simulink model "test"  (R2020b)
settings: Solver=FixedStepDiscrete  StartTime=0.0  StopTime=Inf  RelTol=1e-3
libraries: rpi_blkst x2
settings Model: Creator=jacques  LastModifiedBy=jacques
settings DataIOCC: ReturnWorkspaceOutputs=off
settings OptimizationCC: EnhancedBackFolding=on  PassReuseOutputArgsAs=Individual arguments  ZeroExternalMemoryAtStartup=off  ZeroInternalMemoryAtStartup=off  OptimizeBlockOrder=speed  DifferentSizesBufferReuse=on  OptimizationCustomize=off  EfficientTunableParamExpr=on
settings DebuggingCC: ParameterTunabilityLossMsg=error
settings HardwareCC: ProdBitPerPointer=32  ProdBitPerSizeT=32  ProdBitPerPtrDiffT=32  ProdLargestAtomicInteger=Long  ProdLargestAtomicFloat=Double  ProdWordSize=32  ProdHWDeviceType=ARM Compatible->ARM 11
settings SFSimCC: MATLABDynamicMemAlloc=off
settings RTWCC: Description=RTW Embedded Coder RPI target  SystemTargetFile=ert_rpi.tlc  TemplateMakefile=ert_rpi.tmf  PostCodeGenCommand=postGenFunc(buildInfo)
settings CodeAppCC: ForceParamTrailComments=on  IgnoreCustomStorageClasses=off  OperatorAnnotations=on  SimulinkDataObjDesc=on  SFDataObjDesc=on  InsertBlockDesc=on
settings STFCustomTargetCC: TargetLangStandard=C99 (ISO)  MultiwordLength=256  ModelReferenceCompliant=off  ConcurrentExecutionCompliant=off  CombineOutputUpdateFcns=on  ERTCustomFileBanners=on  SupportNonInlinedSFcns=off  RemoveResetFunc=on  MATLABClassNameForMDSCustomization=Simulink.SoftwareTarget.ERTCustomization  CPPClassGenCompliant=off  GRTInterface=off  SystemTargetFile=ert_rpi.tlc
settings ERTTargetCC: TargetLangStandard=C99 (ISO)  ModelReferenceCompliant=off  ParMdlRefBuildCompliant=off  CompOptLevelCompliant=off  ConcurrentExecutionCompliant=off  SupportContinuousTime=on  ModelStepFunctionPrototypeControlCompliant=off  CPPClassGenCompliant=off  UseToolchainInfoCompliant=off  ExtMode=on  ExtModeMexArgs='10.211.55.9'  ERTCustomFileTemplate=ert_rpi_file_process.tlc

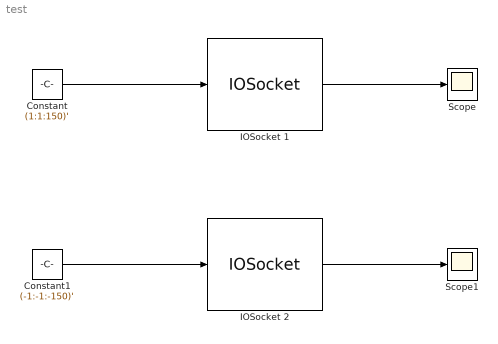
== system test ==
  Constant : Constant  Value=(1:1:150)'  SampleTime=0.05
  Constant1 : Constant  Value=(-1:-1:-150)'  SampleTime=0.05
  IOSocket 1 : rpi_blkst/IOSocket  rpi_mask_Ts=0.005  rpi_mask_ip1=130  rpi_mask_ip2=79  rpi_mask_ip3=245  rpi_mask_ip4=109  rpi_mask_port=31415
      settings: SourceProductName=RPI Blockset
  IOSocket 2 : rpi_blkst/IOSocket  rpi_mask_Ts=0.005  rpi_mask_ip1=130  rpi_mask_ip2=79  rpi_mask_ip3=245  rpi_mask_ip4=109  rpi_mask_port=31416
      settings: SourceProductName=RPI Blockset
  Scope : Scope
  Scope1 : Scope
  wires:
  Constant/1 -> IOSocket 1/1
  Constant1/1 -> IOSocket 2/1
  IOSocket 1/1 -> Scope/1
  IOSocket 2/1 -> Scope1/1
